simulink model "verify_Solar_Collector_basic_mdl"  (R2016b)
settings: Solver=ode45  StartTime=0.0  StopTime=24*3600  MaxStep=100  RelTol=1e-3  EnableMultiTasking=on
libraries: carnot x8, simulink x1
settings Model: Creator=drhf  LastModifiedBy=srrt
settings DataIOCC: LimitDataPoints=on  SaveFormat=Array  SignalLoggingSaveFormat=ModelDataLogs
settings OptimizationCC: ExpressionDepthLimit=2147483647  LifeSpan=inf
settings DebuggingCC: UnderspecifiedInitializationDetection=Classic  MergeDetectMultiDrivingBlocksExec=none  SolverPrmCheckMsg=warning  FcnCallInpInsideContextMsg=warning  StateNameClashWarn=warning  SFUnexpectedBacktrackingDiag=warning  SFNoUnconditionalDefaultTransitionDiag=warning  SFExecutionAtInitializationDiag=none
settings HardwareCC: ProdBitPerPointer=32  ProdBitPerSizeT=32  ProdBitPerPtrDiffT=32  ProdLargestAtomicFloat=None  ProdIntDivRoundTo=Undefined  ProdEndianess=Unspecified  ProdWordSize=32  ProdHWDeviceType=32-bit Generic
settings ModelReferenceCC: PropagateSignalLabelsOutOfModel=off
settings GRTTargetCC: TargetLangStandard=C89/C90 (ANSI)  GeneratePreprocessorConditionals=Disable all  CombineOutputUpdateFcns=off  GRTInterface=on
settings ConfigComp: CovMetricSettings=dw  CovHtmlReporting=on  CovSaveCumulativeToWorkspaceVar=on  CovSaveSingleToWorkspaceVar=on  CovExternalEMLEnable=off

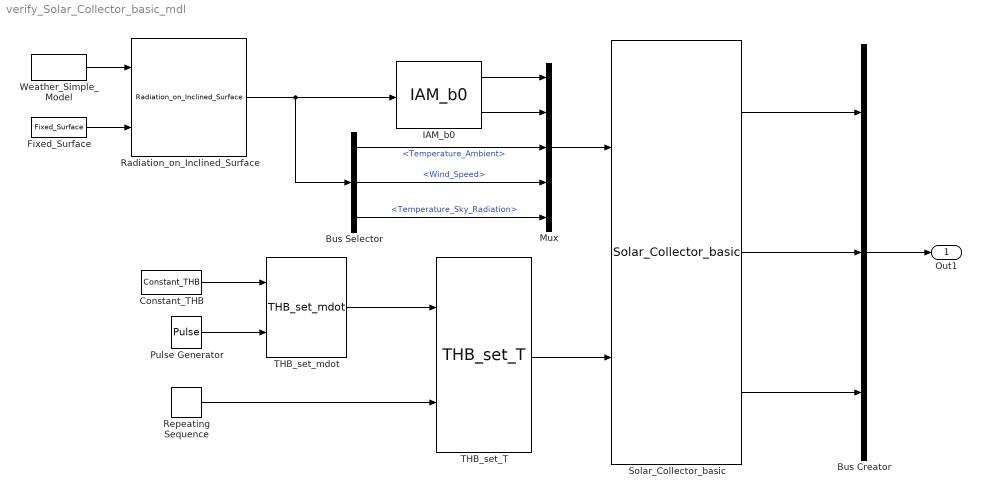
== system verify_Solar_Collector_basic_mdl ==
  Bus Creator : BusCreator  Inputs=3
  Bus Selector : BusSelector  OutputSignals=Temperature_Ambient,Wind_Speed,Temperature_Sky_Radiation
  Constant_THB : carnot/Source/Simple/Constant_THB  t=40  mdot=100/3600  p=1e5  mID=No Pressure Drop  fluid=Water  mix=0  mix2=0  mix3=0  dia=0.02  hgt=0
  Fixed_Surface : carnot/Weather/Fixed_Surface  colangle=30  colazi=0  colrot=0
  IAM_b0 : carnot/Source/Solar_Thermal/IncidenceAngleModifier/IAM_b0  fta=0.8  b0=0.12  Kd=0.92
  Mux : Mux  Inputs=5
  Pulse Generator : DiscretePulseGenerator  PulseType=Time based  Amplitude=100/3600  Period=7*3600  PulseWidth=50
  Radiation_on_Inclined_Surface : carnot/Weather/Radiation_on_Inclined_Surface  sky=Perez 1990  reflect=0.2
  Repeating Sequence : simulink/Sources/Repeating Sequence  rep_seq_t=[0 7 7.1 14 14.1 21 21.1 24]*3600  rep_seq_y=[65 65 75 75 85 85 95 95]
  Solar_Collector_basic : carnot/Basic/Thermal_Models/Solar_Collector_basic  acol=2.5  c1=3.757  c2=0.0147  c3=0  c4=0  c5=7062  c6=0  tini=20
  THB_set_T : carnot/Source/Simple/THB_set_T
  THB_set_mdot : carnot/Source/Simple/THB_set_mdot
  Weather_Simple_Model : carnot/Weather/Weather_Simple_Model  lat=60  Ibn=900  Idg=100  tamb=5  deltaTsky=-6  rh=50  precip="10e-3/24/3600           % 10 mm in 24 h"  cloud=0.125  p=1013e2  vw=1  wdir=270
  Out1 : Outport
  wires:
  Constant_THB/1 -> THB_set_mdot/1
  Pulse Generator/1 -> THB_set_mdot/2
  Bus Creator/1 -> Out1/1
  THB_set_T/1 -> Solar_Collector_basic/2
  THB_set_mdot/1 -> THB_set_T/1
  Repeating Sequence/1 -> THB_set_T/2
  Solar_Collector_basic/2 -> Bus Creator/2
  Solar_Collector_basic/1 -> Bus Creator/1
  Solar_Collector_basic/3 -> Bus Creator/3
  Fixed_Surface/1 -> Radiation_on_Inclined_Surface/2
  Weather_Simple_Model/1 -> Radiation_on_Inclined_Surface/1
  Radiation_on_Inclined_Surface/1 -> Bus Selector/1, IAM_b0/1
  IAM_b0/1 -> Mux/1
  IAM_b0/2 -> Mux/2
  Bus Selector/1 -> Mux/3  "<Temperature_Ambient>"
  Bus Selector/2 -> Mux/4  "<Wind_Speed>"
  Bus Selector/3 -> Mux/5  "<Temperature_Sky_Radiation>"
  Mux/1 -> Solar_Collector_basic/1
